simulink subsystem "DCDCConverterSSC"  (R2023b)
settings: Solver=VariableStepAuto  StartTime=0.0  StopTime=10.0  RelTol=1e-3
undefined symbols (not defined in the file): EnvAirTemp, PlntBattNumCellSer, PlntBattOpenCirctVolt, PlntBattSocInit, PlntBattTempBpt, PlntBattTempInitDegC, PlntBattVoltSocBpt, PlntDCDCEff
libraries: fl_lib x10, ee_lib x1
settings Model: ModifiedByFormat=The MathWorks, Inc.  Creator=The MathWorks, Inc.  LastModifiedBy=The MathWorks, Inc.
settings OptimizationCC: ReuseModelBlockBuffer=off
settings DebuggingCC: SubsystemReferenceDiagnosticForUnitTest=warning

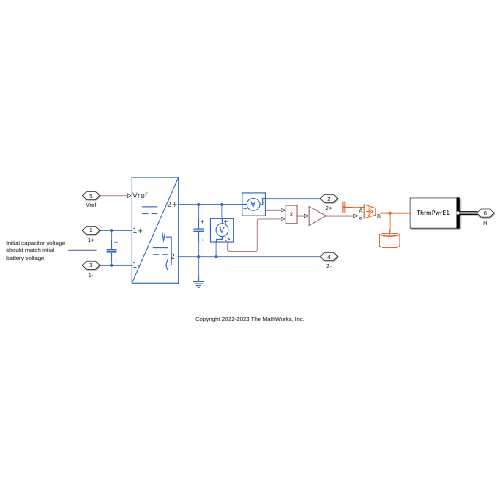
[thumbnail: Simulink's stored preview of the top-level diagram]
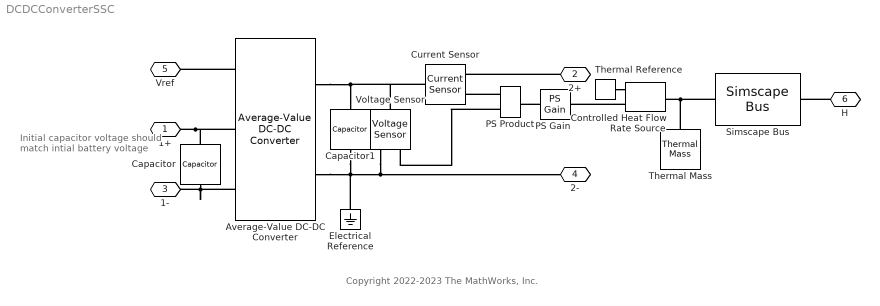
== system DCDCConverterSSC ==
  note: Initial capacitor voltage
      | should match intial
      | battery voltage
  note: Copyright 2022-2023 The MathWorks, Inc.
  Average-Value DC-DC Converter : ee_lib/Semiconductors & Converters/Converters/Average-Value DC-DC Converter  control_option=ee.enum.converters.controlinput.voltage  converter_type=ee.enum.converters.dcdctype.buck  efficiency_option=ee.enum.converters.efficiency.constant  efficiency_fixed=PlntDCDCEff  i_vec=[0, 2, 5] A  efficiency_vec=[90, 95, 98]
      settings: InternalSimscapePortConfiguration="{\"Bottom\":[],\"Left\":[{\"id\":\"Vref\",\"label\":\"Vref\",\"type\":\"input\"},{\"id\":\"p1\",\"label\":\"1+\",\"type\":\"foundation.electrical.electrical\"},{\"id\":\"n1\",\"label\":\"1-\",\"type\":\"foundation.electrical.electrical\"}],\"Right\":[{\"id\":\"p2\",\"label\":\"2+\",\"type\":\"foundation.electrical.electrical\"},{\"id\":\"n2\",\"label\":\"2-\",\"type\":\"foundation.electrical.electrical\"}],\"Top\":[]}"
  Capacitor : fl_lib/Electrical/Electrical Elements/Capacitor  c=PlntDCDCFltrCap uF  r=PlntDCDCFltrRes Ohm  g=0 1/Ohm  i_specify=off  i_priority=None  i=0 A  i_nominal_specify=off  i_nominal_unit=A  i_nominal_value=1  v_specify=off  v_priority=None  v=0 V  v_nominal_specify=off  v_nominal_unit=V  v_nominal_value=1  vc_specify=on  vc_priority=High  vc=interp2(PlntBattTempBpt,PlntBattVoltSocBpt,PlntBattOpenCirctVolt*PlntBattNumCellSer,PlntBattTempInitDegC,PlntBattSocInit) V  vc_nominal_specify=off  vc_nominal_unit=V  vc_nominal_value=1
  Capacitor1 : fl_lib/Electrical/Electrical Elements/Capacitor  c=PlntDCDCFltrCap uF  r=PlntDCDCFltrRes Ohm  g=0 1/Ohm  i_specify=off  i_priority=None  i=0 A  i_nominal_specify=off  i_nominal_unit=A  i_nominal_value=1  v_specify=off  v_priority=None  v=0 V  v_nominal_specify=off  v_nominal_unit=V  v_nominal_value=1  vc_specify=on  vc_priority=High  vc=PlntDCDCVoltInit V  vc_nominal_specify=off  vc_nominal_unit=V  vc_nominal_value=1
  Controlled Heat Flow Rate Source : fl_lib/Thermal/Thermal Sources/Controlled Heat Flow Rate Source
  Current Sensor : fl_lib/Electrical/Electrical Sensors/Current Sensor
  Electrical Reference : fl_lib/Electrical/Electrical Elements/Electrical Reference
  PS Gain : fl_lib/Physical Signals/Functions/PS Gain  gain=(1-PlntDCDCEff/100)/(PlntDCDCEff/100)
  PS Product : fl_lib/Physical Signals/Functions/PS Product
  Simscape Bus : SimscapeBus  HierarchyStrings=ThrmPwrE1
  Thermal Mass : fl_lib/Thermal/Thermal Elements/Thermal Mass  mass_type=foundation.enum.constant_variable.constant  mass=1 kg  sp_heat=385 J/(K*kg)  mass_min=1e-6 kg  num_ports=foundation.enum.numPorts2.one  m_specify=off  m_priority=High  m=1 kg  m_nominal_specify=off  m_nominal_unit=kg  m_nominal_value=1  T_specify=on  T_priority=High  T=EnvAirTemp K  T_nominal_specify=off  T_nominal_unit=K  T_nominal_value=1  Q_specify=off  Q_priority=None  Q=0 W  Q_nominal_specify=off  Q_nominal_unit=W  Q_nominal_value=1
  Thermal Reference : fl_lib/Thermal/Thermal Elements/Thermal Reference
  Voltage Sensor : fl_lib/Electrical/Electrical Sensors/Voltage Sensor
  1+ : PMIOPort  Side=Left
  2+ : PMIOPort  Port=2  Side=Right
  1- : PMIOPort  Port=3  Side=Left
  2- : PMIOPort  Port=4  Side=Right
  Vref : PMIOPort  Port=5  Side=Left
  H : PMIOPort  Port=6  Side=Right
  connections:
  Average-Value DC-DC Converter/RConn1 -- Voltage Sensor/LConn1 -- Current Sensor/LConn1 -- Capacitor1/LConn1
  1+/RConn1 -- Capacitor/LConn1 -- Average-Value DC-DC Converter/LConn2
  Capacitor/RConn1 -- Average-Value DC-DC Converter/LConn3 -- 1-/RConn1
  Capacitor1/RConn1 -- Voltage Sensor/RConn2 -- 2-/RConn1 -- Average-Value DC-DC Converter/RConn2 -- Electrical Reference/LConn1
  Controlled Heat Flow Rate Source/RConn1 -- PS Gain/RConn1
  PS Product/LConn1 -- Current Sensor/RConn1
  PS Product/LConn2 -- Voltage Sensor/RConn1
  PS Gain/LConn1 -- PS Product/RConn1
  Thermal Reference/LConn1 -- Controlled Heat Flow Rate Source/RConn2
  Average-Value DC-DC Converter/LConn1 -- Vref/RConn1
  2+/RConn1 -- Current Sensor/RConn2
  Simscape Bus/LConn1 -- Thermal Mass/LConn1 -- Controlled Heat Flow Rate Source/LConn1
  H/RConn1 -- Simscape Bus/RConn1
